simulink model "Project1"  (R2021a)
settings: Solver=VariableStepAuto  StartTime=0.0  StopTime=0.3  RelTol=1e-3
libraries: fl_lib x15, nesl_utility x8, simulink x2, spsFourierLib x1, ee_lib x1, spsPWMGeneratorDCDCLib x1, eePowerMeasurement x1, eeSinusoidalMeasurementV2 x1, spsTHDLib x1, spspowerguiLib x1
settings Model: Creator=sunchufeng  LastModifiedBy=sunchufeng
settings DataIOCC: ReturnWorkspaceOutputs=off

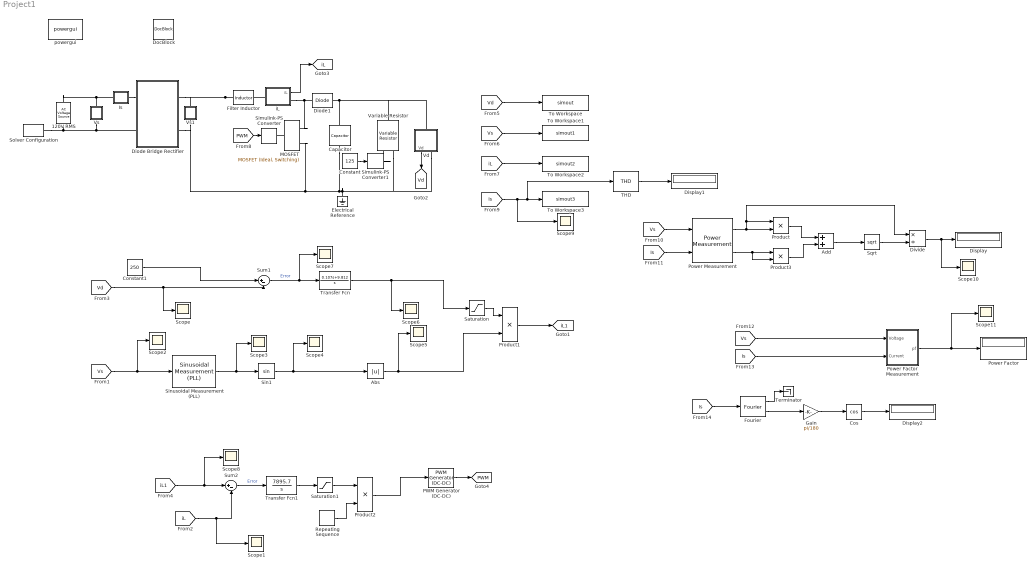
== system Project1 ==
  120V RMS : fl_lib/Electrical/Electrical Sources/AC Voltage Source  amp=120*sqrt(2) V  shift=0 deg  frequency=60 Hz  omega=0 rad/s
  Abs : Abs
  Add : Sum
  Capacitor : fl_lib/Electrical/Electrical Elements/Capacitor  c=200e-6 F  r=200e-6 Ohm  g=0 1/Ohm  i_specify=off  i_priority=None  i=0 A  i_nominal_specify=off  i_nominal_unit=A  i_nominal_value=1  v_specify=off  v_priority=None  v=0 V  v_nominal_specify=off  v_nominal_unit=V  v_nominal_value=1  vc_specify=off  vc_priority=High  vc=0 V  vc_nominal_specify=off  vc_nominal_unit=V  vc_nominal_value=1
  Constant : Constant  Value=125
  Constant1 : Constant  Value=250
  Cos : Trigonometry  Operator=cos
  Diode Bridge Rectifier : Subsystem
  Diode1 : fl_lib/Electrical/Electrical Elements/Diode  Vf=0.6 V  Ron=0.3 Ohm  Goff=1e-8 1/Ohm  i_specify=off  i_priority=None  i=0 A  i_nominal_specify=off  i_nominal_unit=A  i_nominal_value=1  v_specify=off  v_priority=None  v=0 V  v_nominal_specify=off  v_nominal_unit=V  v_nominal_value=1
  Display : Display
  Display1 : Display
  Display2 : Display
  Divide : Product  Inputs=*/
  DocBlock : simulink/Model-Wide Utilities/DocBlock  DocumentType=Text
      content=|
      | This Simulink model demonstrate DC-DC Boost Converter with simple
      | PI Feedback Control to boost 5V DC to 12V DC at switching frequency of 10kHz
  Electrical Reference : fl_lib/Electrical/Electrical Elements/Electrical Reference
  Filter Inductor : fl_lib/Electrical/Electrical Elements/Inductor  l=1.5e-3 H  r=0.01 Ohm  g=1e-9 1/Ohm  i_specify=off  i_priority=None  i=20 A  i_nominal_specify=off  i_nominal_unit=A  i_nominal_value=1  v_specify=off  v_priority=None  v=0 V  v_nominal_specify=off  v_nominal_unit=V  v_nominal_value=1  i_L_specify=off  i_L_priority=High  i_L=0 A  i_L_nominal_specify=off  i_L_nominal_unit=A  i_L_nominal_value=1
  Fourier : spsFourierLib/Fourier  Freq=60  n=1  InInit=[0, 0]  Ts=0
      settings: SourceProductBaseCode=PS
  Gain : Gain  Gain=pi/180
  Is : Subsystem
  MOSFET : ee_lib/Semiconductors & Converters/MOSFET (Ideal, Switching)  Rds=0.01 Ohm  Goff=1e-6 1/Ohm  Vth=0.5 V  diode_param=2  diode_Vf=0.8 V  diode_Ron=0.001 Ohm  diode_Goff=1e-5 1/Ohm  diode_C=5e-8 F  diode_iRM=-235 A  diode_iF=300 A  diode_idot=-50 A/us  diode_trr_param=1  diode_trr_factor=3  diode_trr=15 us  diode_Qrr=1.5e+3 s*uA  thermal_loss_option=ee.enum.converters.thermalLossOption.constantvalues  Von_data=[0, 1.1, 1.3, 1.45, 1.75, 2.25, 2.7; 0, 1, 1.15, 1.35, 1.7, 2.35, 3] V  Eon_data=[0, .29, 1.43, 2.86, 5.71, 13.14, 22.86; 0, .57, 2.63, 5.14, 10.29, 20.57, 30.29] * 1e-3 J  Eoff_data=[0, .21, 1.07, 2.14, 4.29, 9.86, 17.14; 0, .43, 1.97, 3.86, 7.71, 15.43, 22.71] * 1e-3 J  Tj=[298.15, 398.15] K  Iout_data=[0, 10, 50, 100, 200, 400, 600] A  Eon_scalar=22.86e-3 J  Eoff_scalar=17.14e-3 J  Voff=300 V  Iout_scalar=600 A  diodeModelType=ee.enum.converters.diodeModelType.pwl  diode_IfMat=[.07, .12, .19, 1.75, 4.24, 7.32, 11.2; .16, .3, .72, 2.14, 4.02, 6.35, 9.12] A  diode_TjVec=[25, 125] degC  diode_VfVec=[.5, .7, .9, 1.3, 1.7, 2.1, 2.5] V  thermal_network_parameterization=ee.enum.thermalNetworkTopology.external  Rth=[.03, .2] K/W  Rth_Foster=[.03, .2] K/W  thermal_mass_parameterization=ee.enum.thermalNetwork.timeconstant  thermal_mass=[3, 25] J/K  thermal_mass_Foster=[33, 50] J/K  thermal_time_constant=[.1, 5] s  thermal_time_constant_Foster=[1, 10] s  thermal_mass_initial_temperatures=[25, 25] degC  junction_thermal_mass=0.1 J/K  vT_specify=off  vT_priority=None  vT=0 V  vT_nominal_specify=off  vT_nominal_unit=V  vT_nominal_value=1  Qj_specify=off  Qj_priority=None  Qj=0 W  Qj_nominal_specify=off  Qj_nominal_unit=W  Qj_nominal_value=1  junction_temperature_specify=off  junction_temperature_priority=None  junction_temperature=25 degC  junction_temperature_nominal_specify=off  junction_temperature_nominal_unit=degC  junction_temperature_nominal_value=1
  PWM Generator (DC-DC) : spsPWMGeneratorDCDCLib/PWM Generator (DC-DC)  Fsw=100e3  Ts=0
  Power Measurement : eePowerMeasurement/Power Measurement  LabelModeActiveChoice=Continuous  F=60  K=[0 1 2 3]  Ts=0
      settings: SourceProductBaseCode=PS
  Power Factor : Display
  Power Factor Measurement : Subsystem
  Product{,1..3} (4 alike) : Product
  Repeating Sequence : simulink/Sources/Repeating Sequence  rep_seq_t=[0 2]  rep_seq_y=[0 2]
  Saturation : Saturate  UpperLimit=6  LowerLimit=-6
  Saturation1 : Saturate  UpperLimit=6  LowerLimit=-6
  Scope{,1..11} (12 alike) : Scope
  Simulink-PS Converter : nesl_utility/Simulink-PS Converter  PhysicalDomain=network_engine_domain  SubClassName=ps_input  LeftPortType=input  RightPortType=output  PseudoPeriodic=off  Frequencies=[]  NoiseDistribution=none  NoiseParameters=[]  Unit=1  AffineConversion=off  FilteringAndDerivatives=provide  SimscapeFilterOrder=1  InputFilterTimeConstant=0.001  UdotUserProvided=0
  Simulink-PS Converter1 : nesl_utility/Simulink-PS Converter  PhysicalDomain=network_engine_domain  SubClassName=ps_input  LeftPortType=input  RightPortType=output  PseudoPeriodic=off  Frequencies=[]  NoiseDistribution=none  NoiseParameters=[]  Unit=1  AffineConversion=off  FilteringAndDerivatives=provide  SimscapeFilterOrder=1  InputFilterTimeConstant=0.001  UdotUserProvided=0
      settings: SourceProductBaseCode=PW,SS
  Sin1 : Trigonometry
  Sinusoidal Measurement (PLL) : eeSinusoidalMeasurementV2/Sinusoidal Measurement (PLL)  Ki_PD=1000  Kp_LF=400  Ki_LF=20000  F0=60  Theta0=0  Mag0=1  Ts=-1
      settings: SourceProductBaseCode=PS
  Solver Configuration : nesl_utility/Solver Configuration  PhysicalDomain=network_engine_domain  SubClassName=solver  LeftPortType=input  RightPortType=generic  Tones=[]  Harmonics=[]  SimulateNoise=off  Profile=off  UseLocalSampling=off  EnableSwitchedLinearOptims=on  FrequencyDomain=off  UseCCode=off  RelTol=0.001  AbsTol=1e-06  MinStep=1e-09  ToWorkspace=off  RevertToSquareIcSolve=off  NumHomotopyIterations=100  PhasorMode=off  PhasorModeNumHarmonics=1  DoDC=on  ResidualTolerance=1e-09  UseLocalSolver=on  LocalSolverChoice=NE_BACKWARD_EULER_ADVANCER  LocalSolverSampleTime=1/(100*50e3)  DoFixedCost=on  MaxNonlinIter=4  MaxModeIter=2  ComputeImpulses=off  ImpulseIterations=2  LinearAlgebra=Sparse  EquationFormulation=NE_TIME_EF  DelaysMemoryBudget=1024  AutomaticFiltering=on  FilteringTimeConstant=0.001  PartitionStorageMethod=AS_NEEDED  PartitionMemoryBudget=1024  PartitionMethod=FAST
      settings: SourceProductBaseCode=PW,SS
  Sqrt : Sqrt  SaturateOnIntegerOverflow=on
  Sum1 : Sum  Inputs=|+-
  Sum2 : Sum  Inputs=|+-
  THD : spsTHDLib/THD  Freq=60  Ts=0
      settings: SourceProductBaseCode=PS
  Terminator : Terminator
  To Workspace : ToWorkspace  VariableName=simout  SaveFormat=Timeseries  SampleTime=-1
  To Workspace1 : ToWorkspace  VariableName=simout1  SaveFormat=Timeseries  SampleTime=-1
  To Workspace2 : ToWorkspace  VariableName=simout2  SaveFormat=Timeseries  SampleTime=-1
  To Workspace3 : ToWorkspace  VariableName=simout3  SaveFormat=Timeseries  SampleTime=-1
  Transfer Fcn : TransferFcn  Numerator=[0.107 9.812]  Denominator=[1 0]
  Transfer Fcn1 : TransferFcn  Numerator=[7895.7]  Denominator=[1 0]
  Variable Resistor : fl_lib/Electrical/Electrical Elements/Variable Resistor  Rmin=0 Ohm  i_specify=off  i_priority=None  i=0 A  i_nominal_specify=off  i_nominal_unit=A  i_nominal_value=1  v_specify=off  v_priority=None  v=0 V  v_nominal_specify=off  v_nominal_unit=V  v_nominal_value=1
  Vd : Subsystem
  Vs : Subsystem
  Vs1 : Subsystem
  iL : Subsystem
  powergui : spspowerguiLib/powergui  Priority=1  SimulationMode=Discrete  SampleTime=1/10e6  frequency=60  Iterations=50  frequencyindice=0  Pbase=100e6  ErrMax=1e-4  UnitsV=kV  UnitsW=MW  buscounter=0  FunctionMessages=off  echomessages=off  EnableUseOfTLC=off  CurrentSourceSwitches=off  DisableSnubberDevices=off  DisableRonSwitches=off  DisableVfSwitches=off  DisplayEquations=off  AutomaticDiscreteSolvers=off  SolverType=Tustin/Backward Euler (TBE)  Interpol=off  ExternalGateDelay=off  methode=off  Ts=100  x0status=blocks  SPID=off  SwTol=0  HookPort=off  NonlinearTolerance=1e-4  nMaxIteration=100  ContinueOnMaxIteration=off  RestoreLinks=warning  ResistiveCurrentMeasurement=off  Frange=[0:2:500]  Ylog=off  Xlog=on  ShowGrid=off  save=off  variable=ZData  structure=0  ZoomFFT=off  StartTime=0.0  cycles=1  DisplayStyle=1  fundamental=60  FreqAxis=off  MaxFrequency=1000  frequencyindicesteady=1  RmsSteady=1  display=off
  tag scope: PWM=global, Vd=global, iL1=global, iL=global
  wires:
  Constant/1 -> Simulink-PS Converter1/1
  Vd/1(Vd) -> [Vd]
  iL/1(iL) -> [iL]
  Constant1/1 -> Sum1/1
  [Vd] -> Sum1/2, Scope/1
  Sin1/1 -> Abs/1, Scope4/1
  Sum1/1 -> Scope7/1, Transfer Fcn/1  "Error"
  Sum2/1 -> Transfer Fcn1/1  "Error"
  [iL] -> Scope1/1, Sum2/2
  Abs/1 -> Scope5/1, Product1/2
  [Vs] -> Sinusoidal Measurement (PLL)/1, Scope2/1
  Sinusoidal Measurement (PLL)/2 -> Scope3/1, Sin1/1
  Saturation/1 -> Product1/1
  Transfer Fcn/1 -> Scope6/1, Saturation/1
  Transfer Fcn1/1 -> Saturation1/1
  Saturation1/1 -> Product2/1
  Repeating Sequence/1 -> Product2/2
  Product2/1 -> PWM Generator (DC-DC)/1
  Product1/1 -> [iL1]
  [iL1] -> Scope8/1, Sum2/1
  [Vd] -> To Workspace/1
  [Vs] -> To Workspace1/1
  [iL] -> To Workspace2/1
  PWM Generator (DC-DC)/1 -> [PWM]
  [PWM] -> Simulink-PS Converter/1
  [Is] -> Scope9/1, THD/1, To Workspace3/1
  Divide/1 -> Scope10/1, Display/1
  [Vs] -> Power Measurement/1
  [Is] -> Power Measurement/2
  Power Measurement/1 -> Divide/1, Product/1, Product/2
  Power Measurement/2 -> Product3/1, Product3/2
  Product/1 -> Add/1
  Product3/1 -> Add/2
  Add/1 -> Sqrt/1
  Sqrt/1 -> Divide/2
  THD/1 -> Display1/1
  [Is] -> Power Factor Measurement/2(Current)
  [Vs] -> Power Factor Measurement/1(Voltage)
  Power Factor Measurement/1(pf) -> Scope11/1, Power Factor/1
  Fourier/2 -> Gain/1
  [Is] -> Fourier/1
  Gain/1 -> Cos/1
  Cos/1 -> Display2/1
  Fourier/1 -> Terminator/1
  connections:
  Diode Bridge Rectifier/LConn2 -- Vs/RConn1 -- Solver Configuration/RConn1 -- 120V RMS/RConn1
  Capacitor/RConn1 -- Electrical Reference/LConn1 -- Vd/RConn1 -- Variable Resistor/LConn2 -- Vs1/RConn1 -- Diode Bridge Rectifier/RConn2 -- MOSFET/RConn2
  Diode1/RConn1 -- Vd/LConn1 -- Variable Resistor/RConn1 -- Capacitor/LConn1
  iL/RConn1 -- Diode1/LConn1 -- MOSFET/RConn1
  Filter Inductor/LConn1 -- Vs1/LConn1 -- Diode Bridge Rectifier/RConn1
  Simulink-PS Converter1/RConn1 -- Variable Resistor/LConn1
  iL/LConn1 -- Filter Inductor/RConn1
  120V RMS/LConn1 -- Vs/LConn1 -- Is/LConn1
  Simulink-PS Converter/RConn1 -- MOSFET/LConn1
  Is/RConn1 -- Diode Bridge Rectifier/LConn1

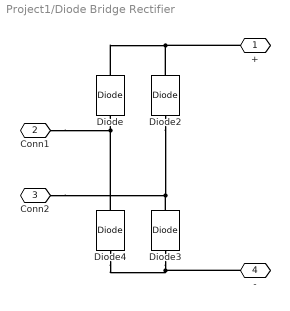
== system Project1/Diode Bridge Rectifier ==
  Diode{,2..4} (4 alike) : fl_lib/Electrical/Electrical Elements/Diode  Vf=0.6 V  Ron=0.3 Ohm  Goff=1e-8 1/Ohm  i_specify=off  i_priority=None  i=0 A  i_nominal_specify=off  i_nominal_unit=A  i_nominal_value=1  v_specify=off  v_priority=None  v=0 V  v_nominal_specify=off  v_nominal_unit=V  v_nominal_value=1
  + : PMIOPort  Side=Right
  Conn1 : PMIOPort  Port=2  Side=Left
  Conn2 : PMIOPort  Port=3  Side=Left
  - : PMIOPort  Port=4  Side=Right
  connections:
  Diode4/LConn1 -- -/RConn1 -- Diode3/LConn1
  Diode/LConn1 -- Conn1/RConn1 -- Diode4/RConn1
  Diode2/RConn1 -- +/RConn1 -- Diode/RConn1
  Diode3/RConn1 -- Conn2/RConn1 -- Diode2/LConn1

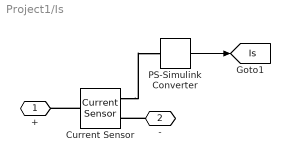
== system Project1/Is ==
  Current Sensor : fl_lib/Electrical/Electrical Sensors/Current Sensor
  PS-Simulink Converter : nesl_utility/PS-Simulink Converter  PhysicalDomain=network_engine_domain  SubClassName=ps_output  LeftPortType=input  RightPortType=output  PseudoPeriodic=off  Frequencies=[]  Unit=1  AffineConversion=off
      settings: SourceProductBaseCode=PW,SS
  + : PMIOPort  Side=Left
  - : PMIOPort  Port=2  Side=Right
  tag scope: Is=global
  wires:
  PS-Simulink Converter/1 -> [Is]
  connections:
  -/RConn1 -- Current Sensor/RConn2
  Current Sensor/RConn1 -- PS-Simulink Converter/LConn1
  Current Sensor/LConn1 -- +/RConn1

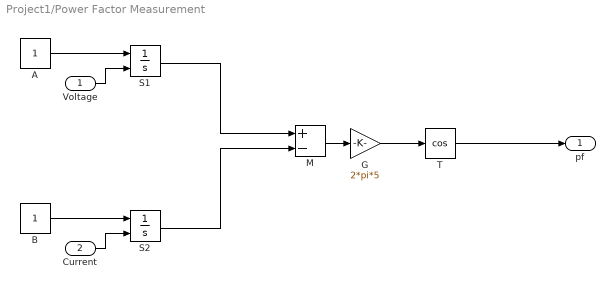
== system Project1/Power Factor Measurement ==
  Voltage : Inport
  Current : Inport  Port=2
  A : Constant
  B : Constant
  G : Gain  Gain=2*pi*5
  M : Sum  Inputs=+-
  S1 : Integrator  ExternalReset=falling
  S2 : Integrator  ExternalReset=falling
  T : Trigonometry  Operator=cos
  pf : Outport
  wires:
  A/1 -> S1/1
  B/1 -> S2/1
  S1/1 -> M/1
  S2/1 -> M/2
  Voltage/1 -> S1/2
  Current/1 -> S2/2
  M/1 -> G/1
  G/1 -> T/1
  T/1 -> pf/1

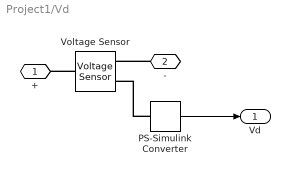
== system Project1/Vd ==
  PS-Simulink Converter : nesl_utility/PS-Simulink Converter  PhysicalDomain=network_engine_domain  SubClassName=ps_output  LeftPortType=input  RightPortType=output  PseudoPeriodic=off  Frequencies=[]  Unit=1  AffineConversion=off
      settings: SourceProductBaseCode=PW,SS
  Voltage Sensor : fl_lib/Electrical/Electrical Sensors/Voltage Sensor
  + : PMIOPort  Side=Left
  - : PMIOPort  Port=2  Side=Right
  Vd : Outport  VectorParamsAs1DForOutWhenUnconnected=off
  wires:
  PS-Simulink Converter/1 -> Vd/1
  connections:
  PS-Simulink Converter/LConn1 -- Voltage Sensor/RConn1
  Voltage Sensor/LConn1 -- +/RConn1
  -/RConn1 -- Voltage Sensor/RConn2

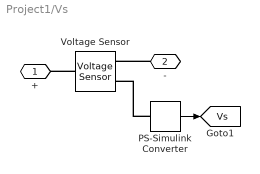
== system Project1/Vs ==
  PS-Simulink Converter : nesl_utility/PS-Simulink Converter  PhysicalDomain=network_engine_domain  SubClassName=ps_output  LeftPortType=input  RightPortType=output  PseudoPeriodic=off  Frequencies=[]  Unit=1  AffineConversion=off
      settings: SourceProductBaseCode=PW,SS
  Voltage Sensor : fl_lib/Electrical/Electrical Sensors/Voltage Sensor
  + : PMIOPort  Side=Left
  - : PMIOPort  Port=2  Side=Right
  tag scope: Vs=global
  wires:
  PS-Simulink Converter/1 -> [Vs]
  connections:
  -/RConn1 -- Voltage Sensor/RConn2
  Voltage Sensor/LConn1 -- +/RConn1
  PS-Simulink Converter/LConn1 -- Voltage Sensor/RConn1

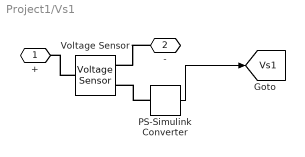
== system Project1/Vs1 ==
  PS-Simulink Converter : nesl_utility/PS-Simulink Converter  PhysicalDomain=network_engine_domain  SubClassName=ps_output  LeftPortType=input  RightPortType=output  PseudoPeriodic=off  Frequencies=[]  Unit=1  AffineConversion=off
      settings: SourceProductBaseCode=PW,SS
  Voltage Sensor : fl_lib/Electrical/Electrical Sensors/Voltage Sensor
  + : PMIOPort  Side=Left
  - : PMIOPort  Port=2  Side=Right
  tag scope: Vs1=global
  wires:
  PS-Simulink Converter/1 -> [Vs1]
  connections:
  PS-Simulink Converter/LConn1 -- Voltage Sensor/RConn1
  Voltage Sensor/LConn1 -- +/RConn1
  -/RConn1 -- Voltage Sensor/RConn2

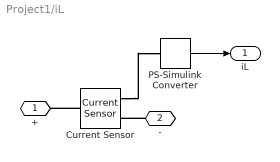
== system Project1/iL ==
  Current Sensor : fl_lib/Electrical/Electrical Sensors/Current Sensor
  PS-Simulink Converter : nesl_utility/PS-Simulink Converter  PhysicalDomain=network_engine_domain  SubClassName=ps_output  LeftPortType=input  RightPortType=output  PseudoPeriodic=off  Frequencies=[]  Unit=1  AffineConversion=off
      settings: SourceProductBaseCode=PW,SS
  + : PMIOPort  Side=Left
  - : PMIOPort  Port=2  Side=Right
  iL : Outport  VectorParamsAs1DForOutWhenUnconnected=off
  wires:
  PS-Simulink Converter/1 -> iL/1
  connections:
  Current Sensor/LConn1 -- +/RConn1
  Current Sensor/RConn1 -- PS-Simulink Converter/LConn1
  -/RConn1 -- Current Sensor/RConn2
